simulink library "xpclib"  (Simulink 6.0)
settings: Solver=ode45  SolverMode=SingleTasking  StartTime=0.0  StopTime=10.0  RelTol=1e-3
values from neighbouring files (symbols this model uses):
  base = get_param( gcb, 'base' )    [maddiamondmm.m]    (also in maddiamondmm32frame.m; maddsmm16at.m; mdadsmm16at.m; mdiortddm64x0.m = hex2dec(addr(3:end)))
  block = find_system(bdroot,                          'FollowLinks', 'on',                          'LookUnderMasks', 'all',                          'MaskType', type )    [mdionipci6527.m]
  count = count + 1    (= 5)    [mdecodestate.m]
  port = get_param( gcb, 'port' )    [mdionipci6527.m]    (also in mdiortddm64x0.m = get_param(blocks{i}, 'port'))
undefined symbols (not defined in the file or in its folder): CIO, devid, DIO24, genixlib, get, handlers, irq, mbaseserialmask, mbwaudpmc, mdacbpcidas, mdiamondemeraldmask, mgenix, mmodemcontrol, mquamask, mrs232, msc150checks, mtargetboxleds, mtargetboxwatchdog, mxpccan, PCI, sizeof, vendid
libraries: xpclib x384, simulink x6
(part 2 of 7)

== system xpclib/A/D ==
  Advantech : Subsystem  PropExecContextAcrossSSBoundary=on
      settings: OpenFcn=load_open_subsystem('xpcadvantechlib','xpcadvantechlib/A//D');
  Analogic : Subsystem  PropExecContextAcrossSSBoundary=on
      settings: OpenFcn=load_open_subsystem('xpcanalogiclib','xpcanalogiclib/A//D');
  Contec : Subsystem  PropExecContextAcrossSSBoundary=on
      settings: OpenFcn=load_open_subsystem('xpcconteclib','xpcconteclib/A//D');
  Data Translation : Subsystem  PropExecContextAcrossSSBoundary=on
      settings: OpenFcn=load_open_subsystem('xpcdatatranslationlib','xpcdatatranslationlib/A//D');
  Diamond : Subsystem  PropExecContextAcrossSSBoundary=on
      settings: OpenFcn=load_open_subsystem('xpcdiamondlib','xpcdiamondlib/A//D');
  General Standards : Subsystem  PropExecContextAcrossSSBoundary=on
      settings: OpenFcn=load_open_subsystem('xpcgeneralstandardslib','xpcgeneralstandardslib/A//D');
  Humusoft : Subsystem  PropExecContextAcrossSSBoundary=on
      settings: OpenFcn=load_open_subsystem('xpchumusoftlib','xpchumusoftlib/A//D');
  Keithley Metrabyte : Subsystem  PropExecContextAcrossSSBoundary=on
      settings: OpenFcn=load_open_subsystem('xpckeithleylib','xpckeithleylib/A//D');
  Measurement Computing : Subsystem  PropExecContextAcrossSSBoundary=on
      settings: OpenFcn=load_open_subsystem('xpcmeasurementcomputinglib','xpcmeasurementcomputinglib/A//D');
  National Instruments : Subsystem  PropExecContextAcrossSSBoundary=on
      settings: OpenFcn=load_open_subsystem('xpcnilib','xpcnilib/A//D');
  Quanser : Subsystem  PropExecContextAcrossSSBoundary=on
      settings: OpenFcn=load_open_subsystem('xpcquanserlib','xpcquanserlib/A//D');
  Real Time Devices : Subsystem  PropExecContextAcrossSSBoundary=on
      settings: OpenFcn=load_open_subsystem('xpcrealtimedeviceslib','xpcrealtimedeviceslib/A//D');
  SBS Technologies : Subsystem  PropExecContextAcrossSSBoundary=on
      settings: OpenFcn=load_open_subsystem('xpcsbstechnologieslib','xpcsbstechnologieslib/A//D');
  Sensoray : Subsystem  PropExecContextAcrossSSBoundary=on
      settings: OpenFcn=load_open_subsystem('xpcsensoraylib','xpcsensoraylib/A//D');
  UEI : Subsystem  PropExecContextAcrossSSBoundary=on
      settings: OpenFcn=load_open_subsystem('xpcueilib','xpcueilib/A//D');
  Versalogic : Subsystem  PropExecContextAcrossSSBoundary=on
      settings: OpenFcn=load_open_subsystem('xpcversalogiclib','xpcversalogiclib/A//D');

== system xpclib/A/D Frame ==
  Diamond : Subsystem  PropExecContextAcrossSSBoundary=on
      settings: OpenFcn=load_open_subsystem('xpcdiamondlib',['xpcdiamondlib/A//D' char(10) 'Frame']);
  UEI : Subsystem  PropExecContextAcrossSSBoundary=on
      settings: OpenFcn=load_open_subsystem('xpcueilib',['xpcueilib/A//D' char(10) 'Frame']);

== system xpclib/Asynchronous Event ==
  Async Buffer Read : S-Function  FunctionName=xpcbuffer  Parameters=DB_Type, sample_time  mask(Asynchronous Buffer Block: Read){sample_time=0.001}
      mask prompts: sample_time "Sample time:"
      mask help: Double Buffer data between asynchronous subsystems/blocks in a model.
      mask init:
      | DB_Type = 'READ';
      mask Help: helpview(fullfile(docroot, 'mapfiles', 'xpc.map'), 'AsynchronousEvent_Async-Buffer-Read')
      mask Display: disp(['xPC Target\nAsynchronous\n Buffer Block\nRead'])
  Async Buffer Write : S-Function  FunctionName=xpcbuffer  Parameters=DB_Type, sample_time  mask(Asynchronous Buffer Block: Write){sample_time=-1}
      mask prompts: sample_time "Sample time:"
      mask help: Double Buffer data between asynchronous subsystems/blocks in a model.
      mask init:
      | DB_Type = 'WRITE';
      mask Help: helpview(fullfile(docroot, 'mapfiles', 'xpc.map'), 'AsynchronousEvent_Async-Buffer-Write')
      mask Display: disp(['xPC Target\nAsynchronous\n Buffer Block\nWrite'])
  Async Rate Transition : Subsystem  PropExecContextAcrossSSBoundary=on  mask(Rate Transition){sample_time=0.001}
      mask prompts: sample_time "Sample time:"
      mask help: Converts rate of input signal to specified sample time.
      mask Help: helpview(fullfile(docroot, 'mapfiles', 'xpc.map'), 'AsynchronousEvent_Async-Rate-Transition')
      mask Display: disp(['xPC Target\nAsynchronous\n Rate\n Transition'])
  IRQ Source : S-Function  FunctionName=xpcinterrupt  Parameters=irq,devid,vendid,slot,handlers,preempt  mask(xpcinterrupt){irqNo=12, preempt=on, b_type=CB CIO-CTR05, slot=-1}
      mask prompts: irqNo "IRQ line number:"; preempt "Allow preemption of function-call subsystem"; b_type "I/O board generating the interrupt:"; slot "PCI slot (-1: autosearch):"
      mask help: Install the downstream function-call subsystem as an xPC Target Interrupt Service Routine.
      mask init:
      | irqNo=irqNo+2;
      | [irq, devid, vendid,slot,handlers] = mxpcinterrupt(irqNo, b_type,slot);
      mask Help: helpview(fullfile(docroot, 'mapfiles', 'xpc.map'), 'AsynchronousEvent_IRQ-Source')
      mask StyleString: popup(3|4|5|6|7|8|9|10|11|12|13|14|15),checkbox,popup(CB CIO-CTR05|CB PCI-CTR05|Softing CAN-AC2-104|Softing CAN-AC2-PCI|RTD DM6804|Audio-PMC+|Scramnet_SC150+|ATI-RP R5|Diamond_MM-32|UEI_MFx|VMIC_5565|SBS_25x0_ID_0x100|SBS_25x0_ID_0x101|SBS_25x0_ID_0x102|SBS_25x0_ID_0x103|None/Other),edit
      mask Display: disp(['xPC Target\nIRQ Source:\n',num2str(irqNo)])

== system xpclib/Audio ==
  Bittware : Subsystem  PropExecContextAcrossSSBoundary=on

== system xpclib/CAN ==
  Softing : Subsystem  PropExecContextAcrossSSBoundary=on
  Utilities : Subsystem  AncestorBlock=xpclib_pc104/CAN/Utilities  PropExecContextAcrossSSBoundary=on

== system xpclib/Counter ==
  Adlink : Subsystem  PropExecContextAcrossSSBoundary=on
      settings: OpenFcn=load_open_subsystem('xpcadlinklib','xpcadlinklib/Counter');
  Diamond : Subsystem  PropExecContextAcrossSSBoundary=on
      settings: OpenFcn=load_open_subsystem('xpcdiamondlib','xpcdiamondlib/Counter');
  Measurement Computing : Subsystem  PropExecContextAcrossSSBoundary=on
      settings: OpenFcn=load_open_subsystem('xpcmeasurementcomputinglib','xpcmeasurementcomputinglib/Counter');
  National Instruments : Subsystem  PropExecContextAcrossSSBoundary=on
      settings: OpenFcn=load_open_subsystem('xpcnilib','xpcnilib/Counter');
  Quanser : Subsystem  PropExecContextAcrossSSBoundary=on
      settings: OpenFcn=load_open_subsystem('xpcquanserlib','xpcquanserlib/Counter');
  Real Time Devices : Subsystem  PropExecContextAcrossSSBoundary=on
      settings: OpenFcn=load_open_subsystem('xpcrealtimedeviceslib','xpcrealtimedeviceslib/Counter');

== system xpclib/D/A ==
  Advantech : Subsystem  PropExecContextAcrossSSBoundary=on
      settings: OpenFcn=load_open_subsystem('xpcadvantechlib','xpcadvantechlib/D//A');
  Contec : Subsystem  PropExecContextAcrossSSBoundary=on
      settings: OpenFcn=load_open_subsystem('xpcconteclib','xpcconteclib/D//A');
  Data Translation : Subsystem  PropExecContextAcrossSSBoundary=on
      settings: OpenFcn=load_open_subsystem('xpcdatatranslationlib','xpcdatatranslationlib/D//A');
  Diamond : Subsystem  PropExecContextAcrossSSBoundary=on
      settings: OpenFcn=load_open_subsystem('xpcdiamondlib','xpcdiamondlib/D//A');
  General Standards : Subsystem  PropExecContextAcrossSSBoundary=on
      settings: OpenFcn=load_open_subsystem('xpcgeneralstandardslib','xpcgeneralstandardslib/D//A');
  Humusoft : Subsystem  PropExecContextAcrossSSBoundary=on
      settings: OpenFcn=load_open_subsystem('xpchumusoftlib','xpchumusoftlib/D//A');
  Keithley Metrabyte : Subsystem  PropExecContextAcrossSSBoundary=on
      settings: OpenFcn=load_open_subsystem('xpckeithleylib','xpckeithleylib/D//A');
  Measurement Computing : Subsystem  PropExecContextAcrossSSBoundary=on
      settings: OpenFcn=load_open_subsystem('xpcmeasurementcomputinglib','xpcmeasurementcomputinglib/D//A');
  National Instruments : Subsystem  PropExecContextAcrossSSBoundary=on
      settings: OpenFcn=load_open_subsystem('xpcnilib','xpcnilib/D//A');
  Quanser : Subsystem  PropExecContextAcrossSSBoundary=on
      settings: OpenFcn=load_open_subsystem('xpcquanserlib','xpcquanserlib/D//A');
  Real Time Devices : Subsystem  PropExecContextAcrossSSBoundary=on
      settings: OpenFcn=load_open_subsystem('xpcrealtimedeviceslib','xpcrealtimedeviceslib/D//A');
  SBS Technologies : Subsystem  PropExecContextAcrossSSBoundary=on
      settings: OpenFcn=load_open_subsystem('xpcsbstechnologieslib','xpcsbstechnologieslib/D//A');
  Sensoray : Subsystem  PropExecContextAcrossSSBoundary=on
      settings: OpenFcn=load_open_subsystem('xpcsensoraylib','xpcsensoraylib/D//A');
  UEI : Subsystem  PropExecContextAcrossSSBoundary=on
      settings: OpenFcn=load_open_subsystem('xpcueilib','xpcueilib/D//A');

== system xpclib/Digital Input ==
  Advantech : Subsystem  PropExecContextAcrossSSBoundary=on
      settings: OpenFcn=load_open_subsystem('xpcadvantechlib',['xpcadvantechlib/Digital' char(10) 'Input']);
  Analogic : Subsystem  PropExecContextAcrossSSBoundary=on
      settings: OpenFcn=load_open_subsystem('xpcanalogiclib',['xpcanalogiclib/Digital' char(10) 'Input']);
  Contec : Subsystem  PropExecContextAcrossSSBoundary=on
      settings: OpenFcn=load_open_subsystem('xpcconteclib',['xpcconteclib/Digital' char(10) 'Input']);
  Data Translation : Subsystem  PropExecContextAcrossSSBoundary=on
      settings: OpenFcn=load_open_subsystem('xpcdatatranslationlib',['xpcdatatranslationlib/Digital' char(10) 'Input']);
  Diamond : Subsystem  PropExecContextAcrossSSBoundary=on
      settings: OpenFcn=load_open_subsystem('xpcdiamondlib',['xpcdiamondlib/Digital' char(10) 'Input']);
  General Standards : Subsystem  PropExecContextAcrossSSBoundary=on
      settings: OpenFcn=load_open_subsystem('xpcgeneralstandardslib',['xpcgeneralstandardslib/Digital' char(10) 'Input']);
  Humusoft : Subsystem  PropExecContextAcrossSSBoundary=on
      settings: OpenFcn=load_open_subsystem('xpchumusoftlib',['xpchumusoftlib/Digital' char(10) 'Input']);
  Keithley Metrabyte : Subsystem  PropExecContextAcrossSSBoundary=on
      settings: OpenFcn=load_open_subsystem('xpckeithleylib',['xpckeithleylib/Digital' char(10) 'Input']);
  Measurement Computing : Subsystem  PropExecContextAcrossSSBoundary=on
      settings: OpenFcn=load_open_subsystem('xpcmeasurementcomputinglib',['xpcmeasurementcomputinglib/Digital' char(10) 'Input']);
  National Instruments : Subsystem  PropExecContextAcrossSSBoundary=on
      settings: OpenFcn=load_open_subsystem('xpcnilib',['xpcnilib/Digital' char(10) 'Input']);
  Quanser : Subsystem  PropExecContextAcrossSSBoundary=on
      settings: OpenFcn=load_open_subsystem('xpcquanserlib',['xpcquanserlib/Digital' char(10) 'Input']);
  Real Time Devices : Subsystem  PropExecContextAcrossSSBoundary=on
      settings: OpenFcn=load_open_subsystem('xpcrealtimedeviceslib',['xpcrealtimedeviceslib/Digital' char(10) 'Input']);
  SBS Technologies : Subsystem  PropExecContextAcrossSSBoundary=on
      settings: OpenFcn=load_open_subsystem('xpcsbstechnologieslib',['xpcsbstechnologieslib/Digital' char(10) 'Input']);
  Sensoray : Subsystem  PropExecContextAcrossSSBoundary=on
      settings: OpenFcn=load_open_subsystem('xpcsensoraylib','xpcsensoraylib/DI');
  UEI : Subsystem  PropExecContextAcrossSSBoundary=on
      settings: OpenFcn=load_open_subsystem('xpcueilib',['xpcueilib/Digital' char(10) 'Input']);
  Versalogic : Subsystem  PropExecContextAcrossSSBoundary=on
      settings: OpenFcn=load_open_subsystem('xpcversalogiclib',['xpcversalogiclib/Digital' char(10) 'Input']);

== system xpclib/Digital Output ==
  Advantech : Subsystem  PropExecContextAcrossSSBoundary=on
      settings: OpenFcn=load_open_subsystem('xpcadvantechlib',['xpcadvantechlib/Digital' char(10) 'Output']);
  Analogic : Subsystem  PropExecContextAcrossSSBoundary=on
      settings: OpenFcn=load_open_subsystem('xpcanalogiclib',['xpcanalogiclib/Digital' char(10) 'Output']);
  Contec : Subsystem  PropExecContextAcrossSSBoundary=on
      settings: OpenFcn=load_open_subsystem('xpcconteclib',['xpcconteclib/Digital' char(10) 'Output']);
  Data Translation : Subsystem  PropExecContextAcrossSSBoundary=on
      settings: OpenFcn=load_open_subsystem('xpcdatatranslationlib',['xpcdatatranslationlib/Digital' char(10) 'Output']);
  Diamond : Subsystem  PropExecContextAcrossSSBoundary=on
      settings: OpenFcn=load_open_subsystem('xpcdiamondlib',['xpcdiamondlib/Digital' char(10) 'Output']);
  General Standards : Subsystem  PropExecContextAcrossSSBoundary=on
      settings: OpenFcn=load_open_subsystem('xpcgeneralstandardslib',['xpcgeneralstandardslib/Digital' char(10) 'Output']);
  Humusoft : Subsystem  PropExecContextAcrossSSBoundary=on
      settings: OpenFcn=load_open_subsystem('xpchumusoftlib',['xpchumusoftlib/Digital' char(10) 'Output']);
  Keithley Metrabyte : Subsystem  PropExecContextAcrossSSBoundary=on
      settings: OpenFcn=load_open_subsystem('xpckeithleylib',['xpckeithleylib/Digital' char(10) 'Output']);
  Measurement Computing : Subsystem  PropExecContextAcrossSSBoundary=on
      settings: OpenFcn=load_open_subsystem('xpcmeasurementcomputinglib',['xpcmeasurementcomputinglib/Digital' char(10) 'Output']);
  National Instruments : Subsystem  PropExecContextAcrossSSBoundary=on
      settings: OpenFcn=load_open_subsystem('xpcnilib',['xpcnilib/Digital' char(10) 'Output']);
  Quanser : Subsystem  PropExecContextAcrossSSBoundary=on
      settings: OpenFcn=load_open_subsystem('xpcquanserlib',['xpcquanserlib/Digital' char(10) 'Output']);
  Real Time Devices : Subsystem  PropExecContextAcrossSSBoundary=on
      settings: OpenFcn=load_open_subsystem('xpcrealtimedeviceslib',['xpcrealtimedeviceslib/Digital' char(10) 'Output']);
  SBS Technologies : Subsystem  PropExecContextAcrossSSBoundary=on
      settings: OpenFcn=load_open_subsystem('xpcsbstechnologieslib',['xpcsbstechnologieslib/Digital' char(10) 'Output']);
  Sensoray : Subsystem  PropExecContextAcrossSSBoundary=on
      settings: OpenFcn=load_open_subsystem('xpcsensoraylib','xpcsensoraylib/DO');
  UEI : Subsystem  PropExecContextAcrossSSBoundary=on
      settings: OpenFcn=load_open_subsystem('xpcueilib',['xpcueilib/Digital' char(10) 'Output']);
  Versalogic : Subsystem  PropExecContextAcrossSSBoundary=on
      settings: OpenFcn=load_open_subsystem('xpcversalogiclib',['xpcversalogiclib/Digital' char(10) 'Output']);

== system xpclib/GPIB ==
  National Instruments : Subsystem  PropExecContextAcrossSSBoundary=on
      settings: OpenFcn=load_open_subsystem('xpcnilib','xpcnilib/GPIB');

== system xpclib/IP Carrier ==
  SBS Technologies : Subsystem  PropExecContextAcrossSSBoundary=on
      settings: OpenFcn=load_open_subsystem('xpcsbstechnologieslib',['xpcsbstechnologieslib/IP' char(10) 'Carrier']);

== system xpclib/Incremental Encoder ==
  ADDI-DATA : Subsystem  PropExecContextAcrossSSBoundary=on
      settings: OpenFcn=load_open_subsystem('xpcaddidatalib',['xpcaddidatalib/Incremental' char(10) 'Encoder']);
  Contec : Subsystem  PropExecContextAcrossSSBoundary=on
      settings: OpenFcn=load_open_subsystem('xpcconteclib',['xpcconteclib/Incremental' char(10) 'Encoder']);
  Measurement Computing : Subsystem  PropExecContextAcrossSSBoundary=on
      settings: OpenFcn=load_open_subsystem('xpcmeasurementcomputinglib',['xpcmeasurementcomputinglib/Incremental' char(10) 'Encoder']);
  National Instruments : Subsystem  PropExecContextAcrossSSBoundary=on
      settings: OpenFcn=load_open_subsystem('xpcnilib',['xpcnilib/Incremental' char(10) 'Encoder']);
  Quanser : Subsystem  PropExecContextAcrossSSBoundary=on
      settings: OpenFcn=load_open_subsystem('xpcquanserlib',['xpcquanserlib/Incremental' char(10) 'Encoder']);
  Real Time Devices : Subsystem  PropExecContextAcrossSSBoundary=on
      settings: OpenFcn=load_open_subsystem('xpcrealtimedeviceslib',['xpcrealtimedeviceslib/Incremental' char(10) 'Encoder']);
  Sensoray : Subsystem  PropExecContextAcrossSSBoundary=on
      settings: OpenFcn=load_open_subsystem('xpcsensoraylib','xpcsensoraylib/Encoder');

== system xpclib/LED ==
  MathWorks : Subsystem  PropExecContextAcrossSSBoundary=on

== system xpclib/LVDT ==
  NAII : Subsystem  PropExecContextAcrossSSBoundary=on
      settings: OpenFcn=load_open_subsystem('xpcnaiilib','xpcnaiilib/LVDT');

== system xpclib/Misc. ==
  From File : S-Function  FunctionName=xpcfromfile  Parameters=filename, dataSize, bufSize, readSize, EOFOption, sampTime  mask(xpcfromfile){filename='', dataSize=8, bufSize=2000, readSize=512, EOFOption=Seek to beginning, sampTime=0.001}
      mask prompts: dataSize "Output port width (bytes):"; bufSize "Buffer size:"; readSize "Disk read size:"; EOFOption "When reaching EOF:"; sampTime "Sample time:"
      mask help: Read data from a file into a software FIFO and output it in real time.
      mask init:
      | EOFOption = EOFOption - 1;
      mask Help: helpview(fullfile(docroot, 'mapfiles', 'xpc.map'), 'Misc_From-File')
      mask StyleString: edit,edit,edit,edit,popup(Hold last output|Seek to beginning),edit
      mask Display: disp('xPC Target\nFrom file')
  "From xPC Target " : Subsystem  PropExecContextAcrossSSBoundary=on  mask(xpc2dng){appname='', blockpath=block, ts=1}
      mask prompts: appname "xPC Target application name:"; blockpath "Signal name (block name):"; ts "Observer sample time:"
      mask init:
      | id=fromxpcmaskinit(appname,blockpath);
      settings: OpenFcn=|
      | try
      | highlightlinexpctag(gcb)
      | catch
      | end
      mask Help: helpview(fullfile(docroot, 'mapfiles', 'xpc.map'), 'Misc_From-xPC-Target')
      mask Display: disp(blockpath);
  "IO port read " : S-Function  FunctionName=xpcportread  Parameters=ports, dtypes, sampletime  mask(xpcportread){port1={'0x300'}, dtype={'uint8'}, sampletime=0.001}
      mask prompts: port1 "I/O port address (cell array):"; dtype "Data type (cell array):"; sampletime "Sample time:"
      mask help:
      | I/O-Port Access
      | Write
      mask init:
      | [ports,maskdisplay, dtypes]=mxpcportio(port1,2, dtype);
      | set_param(gcb,'MaskDisplay',maskdisplay);
      mask Help: helpview(fullfile(docroot, 'mapfiles', 'xpc.map'), 'Misc_IO-port-read')
      mask Display: port_label('output',1,'0x300, 768 ');
  "IO port write " : S-Function  FunctionName=xpcportwrite  Parameters=ports, sampletime  mask(xpcportwrite){port1={'0x300'}, sampletime=0.001}
      mask prompts: port1 "I/O port address (cell array):"; sampletime "Sample time:"
      mask help:
      | I/O-Port Access
      | Write
      mask init:
      | [ports,maskdisplay]=mxpcportio(port1,1);
      | set_param(gcb,'MaskDisplay',maskdisplay);
      mask Help: helpview(fullfile(docroot, 'mapfiles', 'xpc.map'), 'Misc_IO-port-write')
      mask Display: port_label('input',1,' 0x300, 768');
  "Scope (xPC) " : Subsystem  PropExecContextAcrossSSBoundary=on  mask(xpcscopeblock){scopeno=0, scopetype=Target, autostart=on, viewmode=Graphical redraw, formatstr='%15.6f', grid=on, ylimits=[0,0], nosamples=250, noprepostsamples=0, interleave=1, triggermode=FreeRun, triggersignal=1, triggerlevel=0.0, triggerslope=Either, triggerscope=1, triggersample=0, filename=data.dat, mode=Lazy, writesize=512, autorestart=off}
      mask prompts: scopeno "Scope number:"; scopetype "Scope type:"; autostart "Start scope when application starts"; viewmode "Scope mode:"; formatstr "Numerical format:"; ylimits "Y-axis limits:"; nosamples "Number of samples:"; noprepostsamples "Number of pre/post samples:"; triggermode "Trigger mode:"; triggersignal "Trigger signal:"; triggerlevel "Trigger level:"; triggerslope "Trigger slope:"; triggerscope "Trigger scope number:"; triggersample "Sample to trigger on (-1 for end of acquistion):"
      mask init:
      | if scopetype==1
      | scopetypestr='Host';
      | elseif scopetype == 2
      | scopetypestr='Target';
      | elseif scopetype == 3
      | 	scopetypestr = 'File';
      | end
      | modeval = lower(get_param(gcbh, 'Mode'));
      | mxpcscope;
      settings: CopyFcn=incscid
      mask Help: helpview(fullfile(docroot, 'mapfiles', 'xpc.map'), 'Misc_Scope-(xPC)')
      mask StyleString: edit,popup(Host|Target|File),checkbox,popup(Numerical|Graphical redraw|Graphical sliding|Graphical rolling),edit,checkbox,edit,edit,edit,edit,popup(FreeRun|Software triggering|Signal triggering|Scope triggering),edit,edit,popup(Either|Rising|Falling),edit,edit,edit,popup(Lazy|Commit),edit,checkbox
      mask CallbackString: mxpcscope;|mxpcscope||mxpcscope|||||||mxpcscope|||||||||
      mask Display: disp([scopetypestr,' Scope\nId: ',num2str(scopeno)])
  "Software Reboot " : Subsystem  PropExecContextAcrossSSBoundary=on  mask(softwarereboot){sampletime=0.001}
      mask prompts: sampletime "Sample time:"
      mask help:
      | System
      | MotherBoard
      | Software Reboot
      mask Help: helpview(fullfile(docroot, 'mapfiles', 'xpc.map'), 'Misc_Software-Reboot')
      mask Display: disp('System\nMotherBoard');
  "To xPC Target " : Subsystem  PropExecContextAcrossSSBoundary=on  mask(dng2xpc){appname='', blockpath=block, paramname=parameter}
      mask prompts: appname "xPC Target application name:"; blockpath "Path to block in target application:"; paramname "Parameter name:"
      mask init:
      | paramid=toxpcmaskinit(appname,paramname,blockpath);
      settings: OpenFcn=|
      | try
      |     highlightxpctag(gcb)
      | catch
      | end
      mask Help: helpview(fullfile(docroot, 'mapfiles', 'xpc.map'), 'Misc_To-xPC-Target')
      mask Display: disp([blockpath,'\n',paramname]);
  "xPC Target  TET " : S-Function  FunctionName=xpctimeinfo  Parameters=func, ts  mask(xpctet){ts=0.001}
      mask prompts: ts "Sample time:"
      mask help:
      | xPC Target
      | Kernel
      | return current Task Execution Time
      mask init:
      | func=1;
      mask Help: helpview(fullfile(docroot, 'mapfiles', 'xpc.map'), 'Misc_xPC-Target-TET')
      mask Display: disp('TET')
  "xPC Target  Time " : S-Function  FunctionName=xpctimeinfo  Parameters=func, ts  mask(xpctime){ts=0.001}
      mask prompts: ts "Sample time:"
      mask help:
      | xPC Target
      | Kernel
      | return current Kernel time
      mask init:
      | func=2;
      mask Help: helpview(fullfile(docroot, 'mapfiles', 'xpc.map'), 'Misc_xPC-Target-Time')
      mask Display: disp('Time')

== system xpclib/RS232 ==
  note: V1.0 compatible
  note: Composite drivers
  note: Conventional drivers
  "ASCII Decode " : S-Function  FunctionName=asciidecode  Parameters=format, nvars, varids  mask(Asynchronous FIFO Block: reader){format=%d\r, nvars=1, vartypes={ }}
      mask prompts: format "Format string:"; nvars "Number of variables:"; vartypes "Variable types:"
      mask help: FIFO read
      mask init:
      | [ maskdisplay, varids, format ] = masciidecode( 2, format, nvars, vartypes, 1 );
      | set_param( gcb, 'MaskDisplay', maskdisplay );
      mask Help: helpview(fullfile(docroot, 'mapfiles', 'xpc.map'), 'Quatech_ASCII_Decode')
      mask Display: disp( 'ASCII\nDecode');port_label('input',1,'D');port_label('output',1,'1');
  "ASCII Encode " : S-Function  FunctionName=asciiencode  Parameters=format, maxlength, nvars, varids  mask(Ascii Encode){format=%d\r, nvars=1, maxlength=128, vartypes={ 'double' }}
      mask prompts: format "Format string:"; nvars "Number of variables:"; maxlength "Max output string length:"; vartypes "Variable types:"
      mask help: Ascii Encode -- encode input variables as ascii for RS232.
      mask init:
      | [ maskdisplay, varids, format ] = masciidecode( 2, format, nvars, vartypes, 2 );
      | set_param( gcb, 'MaskDisplay', maskdisplay );
      mask Help: helpview(fullfile(docroot, 'mapfiles', 'xpc.map'), 'Quatech_ASCII_Encode')
      mask Display: disp( 'ASCII\nEncode');port_label('output',1,'D');port_label('input',1,'1');
  Asynchronous Mode : Subsystem  PropExecContextAcrossSSBoundary=on
  Binary Mode : Subsystem  PropExecContextAcrossSSBoundary=on
  Diamond : Subsystem  PropExecContextAcrossSSBoundary=on
  "FIFO read " : S-Function  FunctionName=fiforead  Parameters=maxsize, minsize, usedelimiter, delimiter, outputtype, sampletime, enable, enableout  mask(Asynchronous FIFO Block: reader){maxsize=1024, minsize=1, usedelimiter=on, delimiter=13, outputtype=8 bit uint null terminated, enable=off, enableout=off, sampletime=0.001}
      mask prompts: maxsize "Maximum read size:"; minsize "Minimum read size:"; usedelimiter "Read to delimiter:"; outputtype "Output vector type:"; enable "Max and Min read size ports:"; enableout "Enable passthrough:"
      mask help: FIFO read
      mask init:
      | maskdisplay = mfiforw( enable, enableout, 2 );
      | set_param( gcb, 'MaskDisplay', maskdisplay );
      mask Help: helpview(fullfile(docroot, 'mapfiles', 'xpc.map'), 'Quatech_FIFO_Read')
      mask StyleString: edit,edit,checkbox,edit,popup(count+32 bit int|count+32 bit uint|count+16 bit int|count+16 bit uint|8 bit int null terminated|8 bit uint null terminated),checkbox,checkbox,edit
      mask Display: disp( 'FIFO\nRead');port_label('output',1,'D');port_label('input',1,'F');
  "FIFO write " : S-Function  FunctionName=fifowrite  Parameters=size, inputtype, sampletime, present, id  mask(Asynchronous FIFO Block: writer){size=1024, inputtype=8 bit uint null terminated, present=off, sampletime=-1, id=}
      mask prompts: inputtype "Input vector type:"; present "Data present output:"; id "ID (for overflow messages):"
      mask help: FIFO write
      mask init:
      | maskdisplay = mfiforw( present, 0, 1 );
      | set_param(gcb,'MaskDisplay',maskdisplay);
      mask Help: helpview(fullfile(docroot, 'mapfiles', 'xpc.map'), 'Quatech_FIFO_Write')
      mask StyleString: edit,popup(count+32 bit int|count+32 bit uint|count+16 bit int|count+16 bit uint|8 bit int null terminated|8 bit uint null terminated),checkbox,edit,edit
      mask Display: disp( 'FIFO\nwrite');port_label('input',1,'D');port_label('output', 1, 'F');
  Mainboard : Subsystem  PropExecContextAcrossSSBoundary=on
  Quatech : Subsystem  PropExecContextAcrossSSBoundary=on
  "RS232 " : S-Function  InitFcn=mrs232(0);  FunctionName=rs232setup  Parameters=port, baud, dbits, sbits, parity, prot, sbuf, rbuf, 0, istr, iack, iackto, tstr, tack, tackto, initinfo, initackinfo, terminfo, termackinfo  mask(rs232setup){port=COM1, baud=9600, dbits=8, sbits=1, parity=None, prot=None, sbuf=1024, rbuf=1024, initstruct=[], termstruct=[]}
      mask prompts: baud "Baud rate:"; dbits "Number of data bits:"; sbits "Number of stop bits:"; prot "Protocol:"; sbuf "Send buffer size:"; rbuf "Receive buffer size:"; initstruct "Initialization command structure:"; termstruct "Termination command structure:"
      mask help:
      | RS-232
      | Mainboard
      | Setup
      mask init:
      | dmy = '';
      | [istr,iack,dmy,maskdisplay,maskdescription,dmy,dmy,dmy,dmy,initinfo,initackinfo,iackto]=mrs232(2,initstruct,4);
      | [tstr,tack,dmy,maskdisplay,maskdescription,dmy,dmy,dmy,dmy,terminfo,termackinfo,tackto]=mrs232(1,termstruct,4);
      | set_param(gcb,'MaskDisplay',maskdisplay);
      | set_param(gcb,'MaskDescription',maskdescription);
      mask Help: helpview(fullfile(docroot, 'mapfiles', 'xpc.map'), 'RS232_RS232')
      mask StyleString: popup(COM1|COM2|COM3|COM4),popup(115200|57600|38400|19200|9600|4800|2400|1200|600|300|110),popup(8|7),popup(1|2),popup(None|Odd|Even),popup(None|XOn XOff),edit,edit,edit,edit
      mask Display: disp('RS-232\nMainboard\nSetup');
  RS232 State : S-Function  FunctionName=decodestate  Parameters=overrun, parity, frame, breakint, count  mask(RS232 State){overrun=on, parity=on, frame=off, breakint=off}
      mask prompts: overrun "Overrun error output:"; parity "Parity error output"; frame "Framing error output"; breakint "Break interrupt output"
      mask help: RS232 State
      mask init:
      | count = 0;
      | [maskdisplay, count] = mdecodestate( overrun, parity, frame, breakint );
      | set_param( gcb, 'MaskDisplay', maskdisplay );
      mask Help: helpview(fullfile(docroot, 'mapfiles', 'xpc.map'), 'Quatech_State')
      mask Display: disp('RS232\nState');port_label('input',1,'D');port_label('output',1,'D');port_label('output',2,'O');port_label('output',3,'P');
  "Setup " : Subsystem  PropExecContextAcrossSSBoundary=on  mask(rs232setup){port=COM2, baudrate=115200, databit=8, stopbit=1, parity=None, protocol=None, sendbuf=1024, recbuf=1024}
      mask prompts: baudrate "Baud rate:"; databit "Number of data bits:"; stopbit "Number of stop bits:"; sendbuf "Send buffer size:"; recbuf "Receive buffer size:"
      mask Help: helpview(fullfile(docroot,'mapfiles','xpc.map'),'RS232_Setup');
      mask StyleString: popup(COM1|COM2|COM3|COM4),popup(115200|57600|38400|19200|9600|4800|2400|1200|300|110),popup(8|7|6|5),popup(1|2),popup(None|Odd|Even),popup(None|XOnXOff|RTSCTS|DTRDSR),edit,edit
      mask Display: disp('RS232\nMainboard\nSetup');
  Synchronous Mode : Subsystem  PropExecContextAcrossSSBoundary=on

== system xpclib/Shared Memory ==
  Change endianess : S-Function  FunctionName=xpcreverseendian1  Parameters=numInp, lengthIn  mask(xpcreverseendian){numInp=1, lengthIn=Byte}
      mask prompts: numInp "Number of input ports:"; lengthIn "Machine word length:"
      mask Help: helpview(fullfile(docroot, 'mapfiles', 'xpc.map'), 'UDP_Byte-Reversal')
      mask StyleString: edit,popup(Byte|Word|Double Word)
      mask Display: disp('Change\nEndianess')
  SBS Broadcast Memory : Subsystem  PropExecContextAcrossSSBoundary=on
  "Shared Memory Pack " : S-Function  FunctionName=xpcany2dword  Parameters=get(partition(1),'IType'),get(partition(1),'ISize'), get(partition(1),'IAddress'), sizeof(partition(1))  mask(Shared-memory Pack){partition=[]}
      mask prompts: partition "Partition object or structure"
      mask help: Assembles multiple data segments into a continguous block of 32-bit words. The packed data can be written into a shared-memory.
      mask init:
      | partition=smpartition(partition);
      mask Help: helpview(fullfile(docroot, 'mapfiles', 'xpc.map'),'VMIC_5565_Pack')
      mask Display: disp(['pack', char(10), 'Bytes = ' num2str(sizeof(partition))])
  "Shared Memory Unpack " : S-Function  FunctionName=xpcdword2any  Parameters=get(partition(1),'IType'),get(partition(1),'ISize'), get(partition(1),'IAddress'), sizeof(partition(1))  mask(Shared Memory Partition Unpacking){partition=[]}
      mask prompts: partition "Partition object or structure"
      mask help: Extracts multiple data elements from a single packed array of 32-bit words. This is used with 5565 read to define partitions in shared memory.
      mask init:
      | partition=smpartition(partition);
      mask Help: helpview(fullfile(docroot, 'mapfiles', 'xpc.map'),'VMIC_5565_Unpack')
      mask Display: disp(['unpack',char(10),'Bytes = ',num2str(sizeof(partition))])
  Systran : Subsystem  PropExecContextAcrossSSBoundary=on
  VMIC : Subsystem  PropExecContextAcrossSSBoundary=on

== system xpclib/Signal Conditioning ==
  add2 : Subsystem  AncestorBlock=xpclib/Incremental Encoder/ADDI-DATA  PropExecContextAcrossSSBoundary=on

== system xpclib/Synchro Resolver ==
  NAII : Subsystem  PropExecContextAcrossSSBoundary=on
      settings: OpenFcn=load_open_subsystem('xpcnaiilib',['xpcnaiilib/Synchro' char(10) 'Resolver']);
  SBS  Technologies : Subsystem  PropExecContextAcrossSSBoundary=on
      settings: OpenFcn=load_open_subsystem('xpcsbstechnologieslib',['xpcsbstechnologieslib/Synchro' char(10) 'Resolver']);

== system xpclib/Thermo couple ==
  Measurement Computing : Subsystem  PropExecContextAcrossSSBoundary=on
      settings: OpenFcn=load_open_subsystem('xpcmeasurementcomputinglib',['xpcmeasurementcomputinglib/Thermo' char(10) 'couple']);

== system xpclib/UDP ==
  Byte Reversal : S-Function  FunctionName=xpcreverseendian  Parameters=numInp  mask(xpcreverseendian){numInp=1}
      mask prompts: numInp "Number of inputs:"
      mask Help: helpview(fullfile(docroot, 'mapfiles', 'xpc.map'), 'UDP_Byte-Reversal')
      mask Display: disp('Byte\nreversal')
  Pack : S-Function  FunctionName=xpcany2byte  Parameters=datatypesout,byteAlign  mask(xpcany2byte){datatypes={'double'}, byteAlign=1}
      mask prompts: datatypes "Input port datatypes (cell array):"; byteAlign "Byte alignment:"
      mask init:
      | datatypesout= mxpcany2byte(datatypes);
      mask Help: helpview(fullfile(docroot, 'mapfiles', 'xpc.map'), 'UDP_Pack')
      mask StyleString: edit,popup(1|2|4|8)
      mask Display: disp('Pack')
  Receive : S-Function  FunctionName=xpcudpbytereceive  Parameters=ipAddress, ipPort, width, sampletime  mask(xpcudpbytereceive){ipAddress=0.0.0.0, ipPort=25000, width=1, sampletime=0.01}
      mask prompts: ipAddress "IP address to receive from (0.0.0.0 for accepting all):"; ipPort "IP port to receive from:"; width "Output port width (number of bytes):"; sampletime "Sample time:"
      mask Help: helpview(fullfile(docroot, 'mapfiles', 'xpc.map'), 'UDP_Receive')
      mask Display: disp('UDP\nReceive\nBinary')
  Send : S-Function  FunctionName=xpcudpbytesend  Parameters=ipAddress, ipPort, localPort, sampletime  mask(xpcudpbytesend){ipAddress=255.255.255.255, ipPort=25000, localPort=-1, sampletime=0.01}
      mask prompts: ipAddress "IP address to send to (255.255.255.255 for broadcast):"; ipPort "Remote IP port to send to:"; localPort "Use the following local IP port (-1 for automatic port assignment):"; sampletime "Sample time:"
      mask Help: helpview(fullfile(docroot, 'mapfiles', 'xpc.map'), 'UDP_Send')
      mask Display: disp('UDP\nSend\nBinary')
  Unpack : S-Function  FunctionName=xpcbyte2any  Parameters=dimensionsout, datatypesout, byteAlign  mask(xpcbyte2any){dimensions={[1]}, datatypes={'double'}, byteAlign=1}
      mask prompts: dimensions "Output port dimensions (cell array):"; datatypes "Output port datatypes (cell array):"; byteAlign "Byte alignment:"
      mask init:
      | [dimensionsout, datatypesout]= mxpcbyte2any(dimensions, datatypes);
      mask Help: helpview(fullfile(docroot, 'mapfiles', 'xpc.map'), 'UDP_Unpack')
      mask StyleString: edit,edit,popup(1|2|4|8)
      mask Display: disp('Unpack')

== system xpclib/Watchdog ==
  Acces IO : Subsystem  PropExecContextAcrossSSBoundary=on
  MathWorks : Subsystem  PropExecContextAcrossSSBoundary=on
  Versalogic : Subsystem  PropExecContextAcrossSSBoundary=on
      settings: OpenFcn=load_open_subsystem('xpcversalogiclib',['xpcversalogiclib/Watchdog']);

== system xpclib/A/D/Advantech ==

== system xpclib/A/D/Analogic ==

== system xpclib/A/D/Contec ==

== system xpclib/A/D/Data Translation ==

== system xpclib/A/D/Diamond ==

== system xpclib/A/D/General Standards ==

== system xpclib/A/D/Humusoft ==

== system xpclib/A/D/Keithley Metrabyte ==

== system xpclib/A/D/Measurement Computing ==

== system xpclib/A/D/National Instruments ==

== system xpclib/A/D/Quanser ==

== system xpclib/A/D/Real Time Devices ==

== system xpclib/A/D/SBS Technologies ==

== system xpclib/A/D/Sensoray ==

== system xpclib/A/D/UEI ==

== system xpclib/A/D/Versalogic ==

== system xpclib/A/D Frame/Diamond ==

== system xpclib/A/D Frame/UEI ==

== system xpclib/Asynchronous Event/Async Rate Transition ==
  In : Inport  Tag=AsyncRateTransition  SampleTime=sample_time  LatchInput=off
  Out : Outport  Tag=AsyncRateTransition  InitialOutput=0
  wires:
  In/1 -> Out/1

== system xpclib/Audio/Bittware ==
  Audio-PMC+ : S-Function  InitFcn=mbwaudpmc(1)  FunctionName=adbwapmc  Parameters=channel, framesize, samplerate, sampletime, convert, slot  mask(bwaudpmc-ain){channel=[1], framesize=64, samplerate=48000, convert=+-1.000, sampletime=-1, slot=-1}
      mask prompts: channel "Channel Vector:"; framesize "Frame Size (samples):"; samplerate "Sample Rate (Hz):"; convert "Output Format:"; slot "PCI Slot (-1: autosearch):"
      mask help:
      | Audio-PMC+
      | BittWare
      | Analog Input
      mask init:
      | [maskdisplay, framesize, samplerate, sampletime] = mbwaudpmc( 2, channel, framesize, samplerate, sampletime, slot );
      | set_param( gcb, 'MaskDisplay', maskdisplay );
      mask Help: helpview(fullfile(docroot, 'mapfiles', 'xpc.map'), 'BittWare_Audio-PMC_AD')
      mask StyleString: edit,edit,edit,popup(signed 32 bit integer|+-1.000),edit,edit
      mask Display: disp('Audio-PMC\nBittWare\nAnalog Input'); port_label('output',1,'1');
  Audio-PMC+1 : S-Function  InitFcn=mbwaudpmc(1)  FunctionName=dabwapmc  Parameters=channel, framesize, samplerate, sampletime, 0, slot  mask(bwaudpmc-aout){channel=[1], framesize=64, samplerate=48000, sampletime=-1, slot=-1}
      mask prompts: channel "Channel Vector:"; framesize "Frame Size (samples):"; samplerate "Sample Rate (Hz):"; slot "PCI Slot (-1: autosearch):"
      mask help:
      | Audio-PMC+
      | BittWare
      | Analog Output
      mask init:
      | [maskdisplay, framesize, samplerate, sampletime] = mbwaudpmc( 2, channel, framesize, samplerate, sampletime, slot );
      | set_param( gcb, 'MaskDisplay', maskdisplay );
      mask Help: helpview(fullfile(docroot, 'mapfiles', 'xpc.map'), 'BittWare_Audio-PMC_DA')
      mask Display: disp('Audio-PMC\nBittWare\nAnalog Output'); port_label('input',1,'1');

== system xpclib/CAN/Softing ==
  CAN-AC2-104 SJA 1000 : Subsystem  PropExecContextAcrossSSBoundary=on
  CAN-AC2-ISA Intel 527 : Subsystem  PropExecContextAcrossSSBoundary=on
  CAN-AC2-ISA Philips C200 : Subsystem  PropExecContextAcrossSSBoundary=on
  CAN-AC2-PCI SJA 1000 : Subsystem  PropExecContextAcrossSSBoundary=on

== system xpclib/CAN/Utilities ==
  CAN Timeout Detection : Subsystem  AncestorBlock=xpclib_pc104/CAN/Utilities/CAN Timeout Detection  PropExecContextAcrossSSBoundary=on  mask(xpccantimeout){timeout=1}
      mask prompts: timeout "Timeout [s]:"
      mask help:
      | CAN
      | Utilities
      | Timeout Detection
      mask Help: helpview(fullfile(docroot, 'mapfiles', 'xpc.map'), 'Utilities_CAN-Timeout-Detection')
      mask Display: disp(['Timeout = ',num2str(timeout)])
  "CAN bit-packing " : S-Function  AncestorBlock=xpclib_pc104/CAN/Utilities/CAN bit-packing  FunctionName=xpcbit2double  Parameters=bitpatterns, dtypes  mask(bit2double){bitpatterns={ [0:15] }}
      mask prompts: bitpatterns "Bit patterns (cell array):"
      mask help:
      | CAN
      | Utilities
      | Bit-Packing
      mask init:
      | [bitpatterns, dtypes,maskdisplay]=mdoublebit(bitpatterns,[],2);
      | set_param(gcb,'MaskDisplay',maskdisplay);
      mask Help: helpview(fullfile(docroot, 'mapfiles', 'xpc.map'), 'Utilities_CAN-bit-packing')
      mask Display: port_label('input',1,' 0:15');
  "CAN bit-unpacking " : S-Function  AncestorBlock=xpclib_pc104/CAN/Utilities/CAN bit-unpacking  FunctionName=xpcdouble2bit  Parameters=bitpatterns, dtypes  mask(double2bit){bitpatterns={ [0:15] }, dtypes={ 'uint16' }}
      mask prompts: bitpatterns "Bit patterns (cell array):"; dtypes "Data types (cell array):"
      mask help:
      | CAN
      | Utilities
      | Bit-Unpacking
      mask init:
      | [bitpatterns, dtypes, maskdisplay]=mdoublebit(bitpatterns,dtypes,1);
      | set_param(gcb,'MaskDisplay',maskdisplay);
      mask Help: helpview(fullfile(docroot, 'mapfiles', 'xpc.map'), 'Utilities_CAN-bit-unpacking')
      mask Display: port_label('output',1,'0:15 ');

== system xpclib/Counter/Adlink ==

== system xpclib/Counter/Diamond ==

== system xpclib/Counter/Measurement Computing ==

== system xpclib/Counter/National Instruments ==

== system xpclib/Counter/Quanser ==

== system xpclib/Counter/Real Time Devices ==

== system xpclib/D/A/Advantech ==

== system xpclib/D/A/Contec ==

== system xpclib/D/A/Data Translation ==

== system xpclib/D/A/Diamond ==

== system xpclib/D/A/General Standards ==

== system xpclib/D/A/Humusoft ==

== system xpclib/D/A/Keithley Metrabyte ==

== system xpclib/D/A/Measurement Computing ==

== system xpclib/D/A/National Instruments ==

== system xpclib/D/A/Quanser ==

== system xpclib/D/A/Real Time Devices ==

== system xpclib/D/A/SBS Technologies ==

== system xpclib/D/A/Sensoray ==

== system xpclib/D/A/UEI ==

== system xpclib/Digital Input/Advantech ==

== system xpclib/Digital Input/Analogic ==

== system xpclib/Digital Input/Contec ==

== system xpclib/Digital Input/Data Translation ==

== system xpclib/Digital Input/Diamond ==

== system xpclib/Digital Input/General Standards ==

== system xpclib/Digital Input/Humusoft ==

== system xpclib/Digital Input/Keithley Metrabyte ==

== system xpclib/Digital Input/Measurement Computing ==

== system xpclib/Digital Input/National Instruments ==

== system xpclib/Digital Input/Quanser ==

== system xpclib/Digital Input/Real Time Devices ==

== system xpclib/Digital Input/SBS Technologies ==

== system xpclib/Digital Input/Sensoray ==

== system xpclib/Digital Input/UEI ==

== system xpclib/Digital Input/Versalogic ==

== system xpclib/Digital Output/Advantech ==

== system xpclib/Digital Output/Analogic ==

== system xpclib/Digital Output/Contec ==

== system xpclib/Digital Output/Data Translation ==

== system xpclib/Digital Output/Diamond ==

== system xpclib/Digital Output/General Standards ==

== system xpclib/Digital Output/Humusoft ==

== system xpclib/Digital Output/Keithley Metrabyte ==

== system xpclib/Digital Output/Measurement Computing ==

== system xpclib/Digital Output/National Instruments ==

== system xpclib/Digital Output/Quanser ==

== system xpclib/Digital Output/Real Time Devices ==

== system xpclib/Digital Output/SBS Technologies ==

== system xpclib/Digital Output/Sensoray ==

== system xpclib/Digital Output/UEI ==

== system xpclib/Digital Output/Versalogic ==

== system xpclib/GPIB/National Instruments ==

== system xpclib/IP Carrier/SBS Technologies ==

== system xpclib/Incremental Encoder/ADDI-DATA ==

== system xpclib/Incremental Encoder/Contec ==

== system xpclib/Incremental Encoder/Measurement Computing ==

== system xpclib/Incremental Encoder/National Instruments ==

== system xpclib/Incremental Encoder/Quanser ==

== system xpclib/Incremental Encoder/Real Time Devices ==

== system xpclib/Incremental Encoder/Sensoray ==

== system xpclib/LED/MathWorks ==
  "LED " : S-Function  InitFcn=mtargetboxleds(1);  FunctionName=targetboxleds  Parameters=leds, reset, initValue, sampleTime  mask(targetboxleds){leds=[1], reset=[0], initValue=[0], sampleTime=0.001}
      mask prompts: leds "LED vector:"; reset "Reset vector:"; initValue "Initial value vector"; sampleTime "Sample time:"
      mask help:
      | TargetBox 10x120x
      | The MathWorks
      | LED
      mask init:
      | phase = 2;
      | [maskDisplay, maskDescription, reset, initValue] = mtargetboxleds( phase, leds, reset, initValue, sampleTime );
      | set_param(gcb,'MaskDescription',maskDescription);
      | set_param(gcb,'MaskDisplay',maskDisplay);
      mask Help: helpview(fullfile(docroot, 'mapfiles', 'xpc_targetbox.map'), 'TargetBox_LEDs')
      mask Display: disp('TargetBox 10x120x\nThe MathWorks\nLED'); port_label('input', 1, '1');

== system xpclib/LVDT/NAII ==

== system xpclib/Misc./From xPC Target  ==
  xpc2dng : S-Function  AncestorBlock=xpclib/Misc./From xPC Target  FunctionName=xpc2dng  Parameters=ts, id
  Out1 : Outport
  wires:
  xpc2dng/1 -> Out1/1

== system xpclib/Misc./Scope (xPC)  ==
  In1 : Inport  LatchInput=off
  S-Function : S-Function  FunctionName=scblock  Parameters=scopeno, scopetype, viewmode, grid, ylimits, autostart, nosamples, interleave, triggermode, triggersignal, triggerlevel, triggerslope, triggerscope, noprepostsamples,triggersample, filename, modeval, writesize, autorestart,formatstr
  wires:
  In1/1 -> S-Function/1

== system xpclib/Misc./Software Reboot  ==
  In1 : Inport  LatchInput=off
  Data Type  Conversion : DataTypeConversion  OutDataTypeMode=uint8  SaturateOnIntegerOverflow=on  RndMeth=Zero
  Fcn : Fcn  Expr=(u>=0.5)*254
  IO port write1 : S-Function  AncestorBlock=xpclib/Misc./IO port write  FunctionName=xpcportwrite  Parameters=ports, sampletime  mask(xpcportwrite){port1={'0x64'}, sampletime=sampletime}
      mask prompts: port1 "I/O-port address (cell array):"; sampletime "Sample time:"
      mask help:
      | I/O-Port Access
      | Write
      mask init:
      | [ports,maskdisplay]=mxpcportio(port1,1);
      | set_param(gcb,'MaskDisplay',maskdisplay);
      mask Display: port_label('input',1,' 0x64, 100');
  wires:
  In1/1 -> Fcn/1
  Fcn/1 -> Data Type  Conversion/1
  Data Type  Conversion/1 -> IO port write1/1

== system xpclib/Misc./To xPC Target  ==
  In1 : Inport  LatchInput=off
  Data Type Conversion : DataTypeConversion  OutDataTypeMode=double  SaturateOnIntegerOverflow=on  RndMeth=Zero
  IC : InitialCondition
  Memory : Memory
  Relational Operator : RelationalOperator  Operator=~=  InputSameDT=on
  Subsystem : Subsystem  TreatAsAtomicUnit=on  PropExecContextAcrossSSBoundary=on
  wires:
  IC/1 -> Subsystem/Enable
  Relational Operator/1 -> Data Type Conversion/1
  Memory/1 -> Relational Operator/2
  In1/1 -> Subsystem/1(In1), Memory/1, Relational Operator/1
  Data Type Conversion/1 -> IC/1

== system xpclib/RS232/Asynchronous Mode ==
  note: V1.0 compatible
  "RS232 " : S-Function  FunctionName=rs232send  Parameters=port, inStr, inport, numinports, formatsendinfo, ts, waitarg  mask(rs232send){port=COM1, blockvar=[], ts=0.1}
      mask prompts: blockvar "Message struct name:"; ts "Sample time:"
      mask help:
      | RS-232
      | Mainboard
      | Send
      mask init:
      | inStr = '';
      | outStr = '';
      | [inStr,outStr,dtypes,maskdisplay,maskdescription,inport,outport, numinports, numoutports, formatsendinfo, formatrecinfo, waitarg] = mrs232 (1, blockvar, 2);
      | set_param(gcb,'MaskDisplay',maskdisplay);
      | set_param(gcb,'MaskDescription',maskdescription);
      mask Help: helpview(fullfile(docroot, 'mapfiles', 'xpc.map'), 'RS232_Asynchronous-Mode_RS232')
      mask StyleString: popup(COM1|COM2|COM3|COM4),edit,edit
      mask Display: disp('RS-232\nMainboard\nSend');
  RS232 1 : S-Function  FunctionName=rs232rec  Parameters=port, outStr, outport, numoutports, formatrecinfo, dtypes, ts, numeom  mask(rs232rec){port=COM1, blockvar=[], ts=0.1}
      mask prompts: blockvar "Message struct name:"; ts "Sample time:"
      mask help:
      | RS-232
      | Mainboard
      | Receive
      mask init:
      | inStr = '';
      | outStr = '';
      | [inStr,outStr,dtypes,maskdisplay,maskdescription,inport,outport, numinports, numoutports, formatsendinfo, formatrecinfo, waitarg, numeom] = mrs232 (1, blockvar, 1);
      | 
      | 
      | set_param(gcb,'MaskDisplay',maskdisplay);
      | set_param(gcb,'MaskDescription',maskdescription);
      mask Help: helpview(fullfile(docroot, 'mapfiles', 'xpc.map'), 'RS232_Asynchronous-Mode_RS232-1')
      mask StyleString: popup(COM1|COM2|COM3|COM4),edit,edit
      mask Display: disp('RS-232\nMainboard\nReceive');
  "Receive " : Subsystem  PropExecContextAcrossSSBoundary=on  mask(rs232rec){port=COM2, formatrec='start,%f,stop;', numb=1, ts=0.01}
      mask prompts: formatrec "Receive format:"; numb "Number of end-of-message characters:"; ts "Sample time:"
      mask Help: helpview(fullfile(docroot, 'mapfiles', 'xpc.map'), 'RS232_Asynchronous-Mode_Receive')
      mask StyleString: popup(COM1|COM2|COM3|COM4),edit,edit,edit
      mask Display: disp('RS232\nMainboard\nReceive');
  "Send " : Subsystem  PropExecContextAcrossSSBoundary=on  mask(rs232send){port=COM2, formatsend='start,%f,stop;', wait=off, ts=0.01}
      mask prompts: formatsend "Send format:"; wait "Wait until message is transmitted"; ts "Sample time:"
      mask Help: helpview(fullfile(docroot, 'mapfiles', 'xpc.map'), 'RS232_Asynchronous-Mode_Send')
      mask StyleString: popup(COM1|COM2|COM3|COM4),edit,checkbox,edit
      mask Display: disp('RS232\nMainboard\nSend');

== system xpclib/RS232/Binary Mode ==
  Pack : xpclib/UDP/Pack  datatypes={'double'}  byteAlign=1
  RS232 Binary Receive : S-Function  FunctionName=rs232brec  Parameters=port,width,samptime  mask(rs232brec){port=COM1, width=1, samptime=-1}
      mask prompts: port "COM port:"; width "Maximum width per packet:"; samptime "Sample time:"
      mask Help: helpview(fullfile(docroot, 'mapfiles', 'xpc.map'), 'RS232_Binary-Mode_RS232-Binary-Receive')
      mask StyleString: popup(COM1|COM2|COM3|COM4),edit,edit
      mask Display: port_label('input',  1, 'Length');port_label('input',  2, 'Enable');port_label('output', 1, 'Done');port_label('output', 2, 'Data');disp(sprintf('RS232 Receive\nCOM%d', port));
  RS232 Binary Send : S-Function  FunctionName=rs232bsend  Parameters=port,width,samptime  mask(rs232bsend){port=COM1, width=1, samptime=-1}
      mask prompts: port "COM port:"; width "Maximum width per packet:"; samptime "Sample time:"
      mask Help: helpview(fullfile(docroot, 'mapfiles', 'xpc.map'), 'RS232_Binary-Mode_RS232-Binary-Send')
      mask StyleString: popup(COM1|COM2|COM3|COM4),edit,edit
      mask Display: disp(sprintf('RS232 Send\nCOM%d', port));
  Unpack : xpclib/UDP/Unpack  dimensions={[1]}  datatypes={'double'}  byteAlign=1
